simulink model "LoopCounter"  (R2023b)
settings: Solver=VariableStepAuto  StartTime=0.0  StopTime=10.0  RelTol=1e-3
settings Model: Creator=jsonm  LastModifiedBy=jsonm

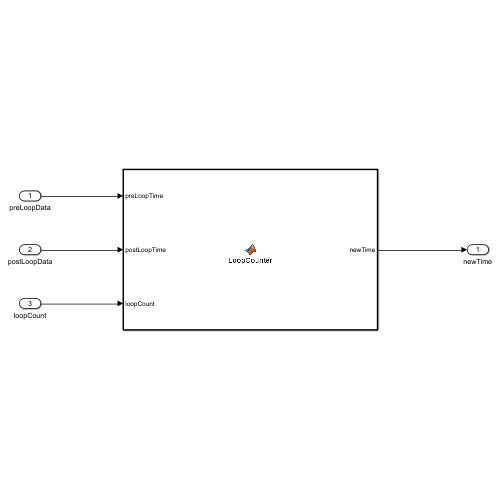
[thumbnail: Simulink's stored preview of the top-level diagram]
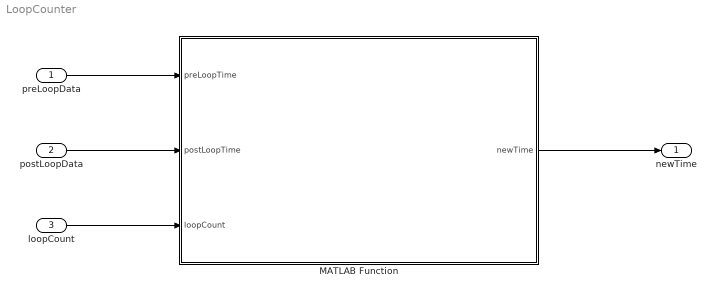
== system LoopCounter ==
  preLoopData : Inport
  postLoopData : Inport  Port=2
  loopCount : Inport  Port=3
  MATLAB Function : MATLAB Function  TreatAsAtomicUnit=on
  newTime : Outport
  wires:
  preLoopData/1 -> MATLAB Function/1(preLoopTime)
  postLoopData/1 -> MATLAB Function/2(postLoopTime)
  loopCount/1 -> MATLAB Function/3(loopCount)
  MATLAB Function/1(newTime) -> newTime/1

== matlab function LoopCounter/MATLAB Function ==
  data: preLoopTime input; newTime output; postLoopTime input; loopCount input
function newTime = LoopCounter(preLoopTime, postLoopTime, loopCount)

% Function to count time generated by loops, assuming each module time has
% been estimated already

newTime = preLoopTime + loopCount*(postLoopTime-preLoopTime);
